simulink model "k_simulink"  (R2013a)
settings: Solver=ode45  StartTime=0.0  StopTime=70  RelTol=1e-3
values from neighbouring files (symbols this model uses):
  Ku = 1/(Q*c*r)    (= 0.00011961722488)    [k_2.m]    (also in k_3.m)
  Q = 2*10^-3    (= 0.002)    [k_2.m]    (also in k_3.m)
  V1 = 10*10^-3    (= 0.01)    [k_2.m]    (also in k_3.m)
  V2 = 14*10^-3    (= 0.014)    [k_2.m]    (also in k_3.m)
  Vr = 4*10^-3    (= 0.004)    [k_2.m]    (also in k_3.m)
libraries: simulink x1
settings Model: Creator=Tobias  LastModifiedBy=Tobias

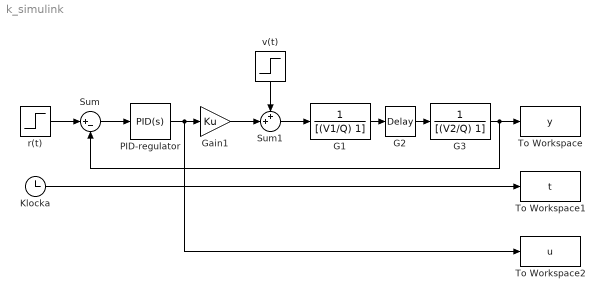
== system k_simulink ==
  G1 : TransferFcn  Denominator=[(V1/Q) 1]
  G2 : TransportDelay  DelayTime=(Vr/Q)  BufferSize=2^20
  G3 : TransferFcn  Denominator=[(V2/Q) 1]
  Gain1 : Gain  Gain=Ku
  Klocka : Clock
  PID-regulator : simulink/Continuous/PID Controller  Controller=PID  TimeDomain=Continuous-time  SampleTime=1  IntegratorMethod=Forward Euler  FilterMethod=Forward Euler  Form=Parallel  P=25194.1165104731  I=1956.14979824376  D=68803.105267141  N=28.6213074510803  InitialConditionSource=internal  InitialConditionForIntegrator=0  InitialConditionForFilter=0  ExternalReset=none  LimitOutput=off  UpperSaturationLimit=inf  LowerSaturationLimit=-inf  LinearizeAsGain=on  AntiWindupMode=none  Kb=1  TrackingMode=off  Kt=1  PParamMin=[]  PParamMax=[]  IParamMin=[]  IParamMax=[]  DParamMin=[]  DParamMax=[]  NParamMin=[]  NParamMax=[]  KbParamMin=[]  KbParamMax=[]  KtParamMin=[]  KtParamMax=[]  POutMin=[]  POutMax=[]  IOutMin=[]  IOutMax=[]  DOutMin=[]  DOutMax=[]  NOutMin=[]  NOutMax=[]  KbOutMin=[]  KbOutMax=[]  KtOutMin=[]  KtOutMax=[]  IntegratorOutMin=[]  IntegratorOutMax=[]  FilterOutMin=[]  FilterOutMax=[]  SumOutMin=[]  SumOutMax=[]  SumI1OutMin=[]  SumI1OutMax=[]  SumI2OutMin=[]  SumI2OutMax=[]  SumI3OutMin=[]  SumI3OutMax=[]  SumDOutMin=[]  SumDOutMax=[]  SaturationOutMin=[]  SaturationOutMax=[]  IntegratorContinuousStateAttributes=''  IntegratorStateMustResolveToSignalObject=off  IntegratorRTWStateStorageClass=Auto  FilterContinuousStateAttributes=''  FilterStateMustResolveToSignalObject=off  FilterRTWStateStorageClass=Auto
  Sum : Sum  Inputs=|+-
  Sum1 : Sum  Inputs=++|
  To Workspace : ToWorkspace  VariableName=y  SampleTime=-1
  To Workspace1 : ToWorkspace  VariableName=t  SampleTime=-1
  To Workspace2 : ToWorkspace  VariableName=u  SampleTime=-1
  r(t) : Step  After=0  SampleTime=1
  v(t) : Step  After=-1  SampleTime=1
  wires:
  G1/1 -> G2/1
  G2/1 -> G3/1
  Sum1/1 -> G1/1
  PID-regulator/1 -> To Workspace2/1, Gain1/1
  Sum/1 -> PID-regulator/1
  Klocka/1 -> To Workspace1/1
  Gain1/1 -> Sum1/2
  r(t)/1 -> Sum/1
  G3/1 -> Sum/2, To Workspace/1
  v(t)/1 -> Sum1/1
